simulink model "FIR_1GHz_4CH"  (R2020b)
settings: Solver=VariableStepAuto  StartTime=0.0  StopTime=10.0  RelTol=1e-3
libraries: xbsIndex_r4 x16, dspsigops x4, dspsrcs4 x2
settings Model: Creator=ehsan.roshanshomal  LastModifiedBy=ehsan.roshanshomal

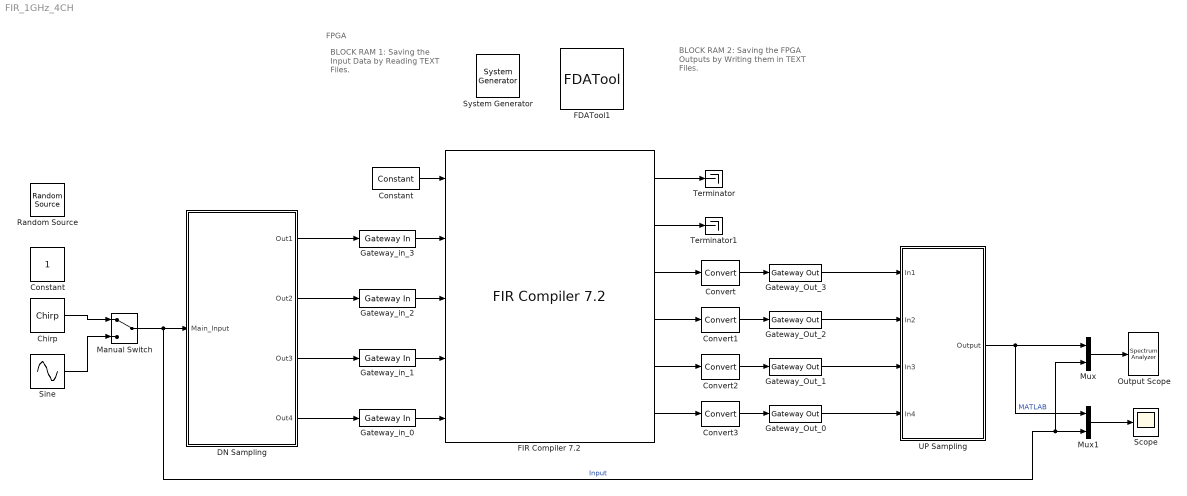
== system FIR_1GHz_4CH ==
  note: BLOCK RAM 1:
      |
      | Saving the Input
      | Data by Reading
      | TEXT Files.
  note: FPGA
  note: BLOCK RAM 2:
      |
      | Saving the FPGA
      | Outputs by Writing
      | them in TEXT Files.
  " System Generator" : xbsIndex_r4/ System Generator  Tag=genX  xilinxfamily=spartan7  part=xc7s50  speed=-1  package=csga324  synthesis_tool=Vivado  clock_wrapper=Clock Enables  directory=./netlist  proj_type=Vivado  Synth_file=Vivado Synthesis Defaults  Impl_file=Vivado Implementation Defaults  testbench=off  simulink_period=1/250e6  sysclk_period=4  dcm_input_clock_period=10  incr_netlist=off  trim_vbits=Everywhere in SubSystem  dbl_ovrd=According to Block Masks  core_generation=According to Block Masks  run_coregen=off  deprecated_control=off  eval_field=0  block_type=sysgen
  Chirp : dspsrcs4/Chirp  sweep=Swept cosine  mode=Bidirectional  f0=0  f1=20e9  t1=0.05  Tsweep=0.25  phase=0  Ts=1/1e9  spf=1  datatype=Double  OutputFrames=off
  Constant : Constant  SampleTime=1/1e9
  "Constant " : xbsIndex_r4/Constant  const=1.0  gui_display_data_type=Boolean  arith_type=Boolean  n_bits=16  bin_pt=14  preci_type=Single  exp_width=8  frac_width=24  explicit_period=on  period=1/250e6  equ=P=C  opselect=C  inp2=PCIN>>17  opr=+  inp1=P  carry=CIN  dbl_ovrd=off  block_type=constant
  Convert{,1..3} (4 alike) : xbsIndex_r4/Convert  gui_display_data_type=Fixed-point  arith_type="Signed  (2's comp)"  n_bits=14  bin_pt=12  float_type=Single  exp_bits=8  fraction_bits=24  quantization=Truncate  overflow=Wrap  en=off  latency=0  pipeline=off  dbl_ovrd=off  block_type=convert
  DN Sampling : Subsystem
  FDATool1 : xbsIndex_r4/FDATool  block_type=fdatool
      settings: infoedit=FDATool
  FIR Compiler 7.2 : xbsIndex_r4/FIR Compiler 7.2   coefficientvector=[0.04799215931962855924419741882047674153,0.018199518094133202567030949126092309598,-0.12670391152623003416799463138886494562,0.250814987351776430557492858497425913811,0.694152403244554516703601620974950492382,0.250814987351776430557492858497425913811,-0.12670391152623003416799463138886494562,0.018199518094133202567030949126092309598,0.04799215931962855924419741882047674153]  coefficient_sets=1  coefficient_reload=off  filter_type=Single_Rate  rate_change_type=Integer  interpolation_rate=1  decimation_rate=1  zero_pack_factor=1  channel_sequence=Basic  number_channels=1  pattern_list='P4-0,P4-1,P4-2,P4-3,P4-4'  number_paths=1  ratespecification=Input_Sample_Period  sampleperiod=0.25000000  hardwareoversamplingrate=1  coefficient_sign=Signed  quantization=Quantize_Only  coefficient_width=12  bestprecision=off  coefficient_fractional_bits=11  coefficient_structure=Inferred  output_rounding_mode=Full_Precision  output_width=28  filter_architecture=Systolic_Multiply_Accumulate  optimization_goal=Area  optimization_list='None'  data_buffer_type=Automatic  coefficient_buffer_type=Automatic  input_buffer_type=Automatic  output_buffer_type=Automatic  preference_for_other_storage=Automatic  multi_column_support=Automatic  columnconfig='5'  inter_column_pipe_length=4  data_has_tlast=Not_Required  m_data_has_tready=off  s_data_has_fifo=off  s_data_has_tuser=Not_Required  m_data_has_tuser=Not_Required  s_config_sync_mode=On_Vector  s_config_method=Single  num_reload_slots=1  has_aclken=off  has_aresetn=off  infoeditControl=ARESETn must be asserted for a minimum of 2 cycles  reset_data_vector=on  trim_axipin_name=on  simulation_type=hybrid_sim  simulation_model=sysgen:xfirv7_2_cmodel  data_path_portlist={ 's_axis_data_tdata', 'm_axis_data_tdata' }  passband_min=0.0  passband_max=0.5  stopband_min=0.5  stopband_max=1.0  filter_selection=1  gui_behaviour='Sysgen_GUI'  data_sign=Signed  data_width=16  data_fractional_bits=0  data_tuser_width=1  wrapper_available=true  ip_wrap_arbitrary_binary_point=true  ip_name=FIR Compiler  ip_version=7.2  dsptool_ready=true  ipcore_usecache=true  ipcore_useipmodelcache=true  port_translation_map={ 'aclken' => 'en', 'aresetn' => 'rst' }  run_core_at_system_period=true  ipcore_xco_need_fpga_part=true  block_type=fir_compiler_v7_2
      settings: infoedit=Maximum Possible : Maximizes oversampling rate. Abstracted input handshake (no s_data_tvalid) and automatic rate propagation.<br>Hardware Oversampling Rate : Specifies oversampling rate relative to the input sample period. Abstracted input handshake (no s_data_tvalid) and automatic rate propagation.<br>Input/Output Sample Period : Specifies absolute oversampling rate. No input handshake abstraction (exposes s_data_tvalid) and no rate propagation.
  Gateway_Out_{0..3} (4 alike) : xbsIndex_r4/Gateway Out  inherit_from_input=off  hdl_port=on  rows=1  columns=1  UseAsDAC=off  DACChannel='1'  interface=None  automatic_assignment=on  address_offset=hex2dec('00')  intf_name=''  intf_description=''  timing_constraint=None  locs_specified=off  LOCs={}  io_standard={}  block_type=gatewayout
  Gateway_in_{0..3} (4 alike) : xbsIndex_r4/Gateway In  gui_display_data_type=Fixed-point  arith_type="Signed  (2's comp)"  n_bits=14  bin_pt=12  preci_type=Single  exp_width=8  frac_width=24  rows=1  columns=1  quantization="Round  (unbiased: +/- Inf)"  overflow=Saturate  period=1/250e6  UseAsADC=off  ADCChannel='1'  interface=None  automatic_assignment=on  address_offset=hex2dec('00')  intf_name=''  intf_description=''  default_value=0  timing_constraint=None  locs_specified=off  LOCs={}  io_standard={}  inherit_from_input=off  hdl_port=on  dbl_ovrd=off  block_type=gatewayin
  Manual Switch : ManualSwitch
  Mux : Mux  Inputs=2
  Mux1 : Mux  Inputs=2
  Output Scope : SpectrumAnalyzer
  "Random Source " : dspsrcs4/Random Source  SrcType=Uniform  NormMethod=Ziggurat  CltLength=12  MinVal=0  MaxVal=0.99  MeanVal=0  VarVal=1  RepMode=Not repeatable  rawSeed=1  IsInherit=off  SampMode=Discrete  SampTime=1/1e9  SampFrame=1  DataType=Double  OutComplex=Real  OutputFrames=off
  Scope : Scope
  Sine : Sin  Frequency=2*pi*53e6  SampleTime=1/1e9  VectorParams1D=off
  Terminator : Terminator
  Terminator1 : Terminator
  UP Sampling : Subsystem
  wires:
  Gateway_in_3/1 -> FIR Compiler 7.2/2
  Gateway_in_2/1 -> FIR Compiler 7.2/3
  Gateway_in_1/1 -> FIR Compiler 7.2/4
  Gateway_in_0/1 -> FIR Compiler 7.2/5
  FIR Compiler 7.2/3 -> Convert/1
  "Constant "/1 -> FIR Compiler 7.2/1
  FIR Compiler 7.2/4 -> Convert1/1
  FIR Compiler 7.2/5 -> Convert2/1
  FIR Compiler 7.2/6 -> Convert3/1
  FIR Compiler 7.2/1 -> Terminator/1
  FIR Compiler 7.2/2 -> Terminator1/1
  Convert/1 -> Gateway_Out_3/1
  Convert1/1 -> Gateway_Out_2/1
  Convert2/1 -> Gateway_Out_1/1
  Convert3/1 -> Gateway_Out_0/1
  Sine/1 -> Manual Switch/2
  Mux/1 -> Output Scope/1
  Mux1/1 -> Scope/1
  Manual Switch/1 -> Mux1/2, Mux/2, DN Sampling/1(Main_Input)  "Input"
  DN Sampling/1(Out1) -> Gateway_in_3/1
  DN Sampling/2(Out2) -> Gateway_in_2/1
  DN Sampling/3(Out3) -> Gateway_in_1/1
  DN Sampling/4(Out4) -> Gateway_in_0/1
  Gateway_Out_3/1 -> UP Sampling/1(In1)
  Gateway_Out_2/1 -> UP Sampling/2(In2)
  Gateway_Out_1/1 -> UP Sampling/3(In3)
  Gateway_Out_0/1 -> UP Sampling/4(In4)
  UP Sampling/1(Output) -> Mux1/1, Mux/1  "MATLAB"
  Chirp/1 -> Manual Switch/1

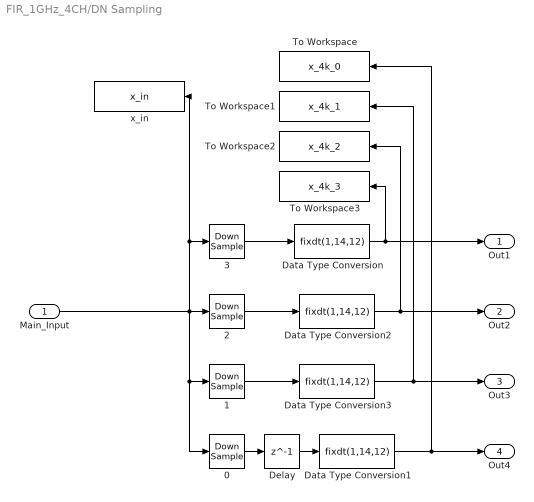
== system FIR_1GHz_4CH/DN Sampling ==
  Main_Input : Inport
  0 : DownSample  N=4  RateOptions=Allow multirate processing
  1 : DownSample  N=4  phase=1  RateOptions=Allow multirate processing
  2 : DownSample  N=4  phase=2  RateOptions=Allow multirate processing
  3 : DownSample  N=4  phase=3  RateOptions=Allow multirate processing
  Data Type Conversion{,1..3} (4 alike) : DataTypeConversion  OutDataTypeStr=fixdt(1,14,12)
  Delay : Delay  DelayLength=1
  To Workspace : ToWorkspace  VariableName=x_4k_0  SampleTime=-1
      settings: Save2DSignal=2-D array (concatenate along first dimension)
  To Workspace1 : ToWorkspace  VariableName=x_4k_1  SampleTime=-1
      settings: Save2DSignal=2-D array (concatenate along first dimension)
  To Workspace2 : ToWorkspace  VariableName=x_4k_2  SampleTime=-1
      settings: Save2DSignal=2-D array (concatenate along first dimension)
  To Workspace3 : ToWorkspace  VariableName=x_4k_3  SampleTime=-1
      settings: Save2DSignal=2-D array (concatenate along first dimension)
  x_in : ToWorkspace  VariableName=x_in  SampleTime=-1
      settings: Save2DSignal=2-D array (concatenate along first dimension)
  Out1 : Outport
  Out2 : Outport  Port=2
  Out3 : Outport  Port=3
  Out4 : Outport  Port=4
  wires:
  Delay/1 -> Data Type Conversion1/1
  3/1 -> Data Type Conversion/1
  2/1 -> Data Type Conversion2/1
  1/1 -> Data Type Conversion3/1
  0/1 -> Delay/1
  Data Type Conversion1/1 -> Out4/1, To Workspace/1
  Main_Input/1 -> 0/1, 1/1, x_in/1, 3/1, 2/1
  Data Type Conversion3/1 -> Out3/1, To Workspace1/1
  Data Type Conversion2/1 -> Out2/1, To Workspace2/1
  Data Type Conversion/1 -> Out1/1, To Workspace3/1

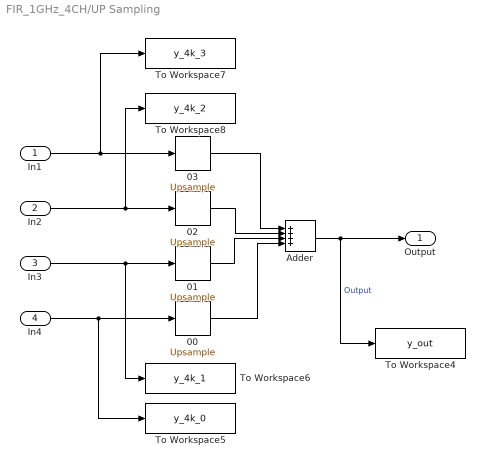
== system FIR_1GHz_4CH/UP Sampling ==
  In1 : Inport
  In2 : Inport  Port=2
  In3 : Inport  Port=3
  In4 : Inport  Port=4
  00 : dspsigops/Upsample  N=4  phase=0  RateOptions=Allow multirate processing  ic=0  mode=Unused parameter value
  01 : dspsigops/Upsample  N=4  phase=1  RateOptions=Allow multirate processing  ic=0  mode=Unused parameter value
  02 : dspsigops/Upsample  N=4  phase=2  RateOptions=Allow multirate processing  ic=0  mode=Unused parameter value
  03 : dspsigops/Upsample  N=4  phase=3  RateOptions=Allow multirate processing  ic=0  mode=Unused parameter value
  Adder : Sum  Inputs=++++
  To Workspace4 : ToWorkspace  VariableName=y_out  SampleTime=-1
      settings: Save2DSignal=2-D array (concatenate along first dimension)
  To Workspace5 : ToWorkspace  VariableName=y_4k_0  SampleTime=-1
      settings: Save2DSignal=2-D array (concatenate along first dimension)
  To Workspace6 : ToWorkspace  VariableName=y_4k_1  SampleTime=-1
      settings: Save2DSignal=2-D array (concatenate along first dimension)
  To Workspace7 : ToWorkspace  VariableName=y_4k_3  SampleTime=-1
      settings: Save2DSignal=2-D array (concatenate along first dimension)
  To Workspace8 : ToWorkspace  VariableName=y_4k_2  SampleTime=-1
      settings: Save2DSignal=2-D array (concatenate along first dimension)
  Output : Outport
  wires:
  In1/1 -> To Workspace7/1, 03/1
  02/1 -> Adder/2
  03/1 -> Adder/1
  In4/1 -> To Workspace5/1, 00/1
  In2/1 -> 02/1, To Workspace8/1
  In3/1 -> To Workspace6/1, 01/1
  00/1 -> Adder/4
  01/1 -> Adder/3
  Adder/1 -> Output/1, To Workspace4/1  "Output"
